simulink model "simulink_6"  (R2017a)
settings: Solver=VariableStepAuto  StartTime=0.0  StopTime=10.0  RelTol=1e-3
values from neighbouring files (symbols this model uses):
  C_d = c2d(tf(C),Tc,'tustin')    [es6.m]
  sys_c = tf(num_c,den_c)    [es6.m]
  Tc = 2*pi/500    (= 0.0125663706144)    [es6.m]
settings Model: Creator=Umberto  LastModifiedBy=Umberto

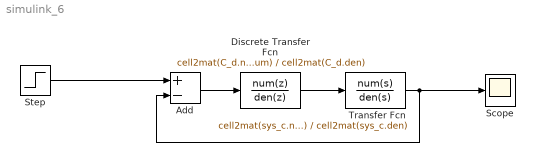
== system simulink_6 ==
  Add : Sum  Inputs=+-
  Discrete Transfer Fcn : DiscreteTransferFcn  Numerator=cell2mat(C_d.num)  Denominator=cell2mat(C_d.den)  SampleTime=Tc
  Scope : Scope
  Step : Step  SampleTime=0
  Transfer Fcn : TransferFcn  Numerator=cell2mat(sys_c.num)  Denominator=cell2mat(sys_c.den)
  wires:
  Discrete Transfer Fcn/1 -> Transfer Fcn/1
  Add/1 -> Discrete Transfer Fcn/1
  Transfer Fcn/1 -> Add/2, Scope/1
  Step/1 -> Add/1
